simulink model "Appl_DrLearn_CtrlModel"  (R2018b)
settings: configuration reference "CodeConfig_10_ms" (kept outside this file)
undefined symbols (not defined in the file): CAL_LearnAllTimeMax_150s, CAL_LearnSingleTimeMax_60s, D_FirstMove, D_FourthlyMove, D_Invalid, D_SecondMove, D_ThirdlyMove, enDrAdjustEnable, FALSE, TRUE
libraries: DareLib x43, simulink x2
(part 2 of 2)

== stateflow chart Appl_DrLearn_CtrlModel/LogicCtrl/LocalAdjustCtrl/LearnReqDeal/Learn ==
  state [Hight,H_Move,Length,L_Move,Back,B_Move,Front,F_Move] = MotorLearnOrderPrm(VehicleTypePrm) [function] [commented out]
  state SetDescLearnStsForDebug(Sts) [function] [commented out]
  state SetDescLearnSts(Sts) [function]
  note: /*Hight,H_Move,Length,L_Move,Back,B_Move,Front,F_Move = MotorLearnOrderPrm(MtrCtrl_VehiclePrm);*/
  state Init
    en:
    SetDescLearnSts(FALSE);
    HeightLearnSW = enNULL;
    LengthLearnSW = enNULL;
    BackLearnSW = enNULL;
    FrontLearnSW = enNULL;;
    LearnResult = 0;
    MotorMtrCtrl_LearnSts = 0;
    Hight =D_FirstMove;
    H_Move =  enDOWN_BACK;
    Length =  D_SecondMove;
    L_Move = enUP_FORWARD;
    Back =  D_ThirdlyMove;
    B_Move = enUP_FORWARD;
    Front = D_FourthlyMove;
    F_Move = enUP_FORWARD;
  state LearnReady
    en:
    SetDescLearnSts(FALSE);
    HeightLearnSW = enNULL;
    LengthLearnSW = enNULL;
    BackLearnSW = enNULL;
    FrontLearnSW = enNULL;;
    LearnResult = 0;
    MotorMtrCtrl_LearnSts = 0;
    (default) -> (junction 223)
    LearnReady -> (junction 223) [order 1]
    (junction 223) -> (junction 225) [order 1] : [MtrCtrl_AdjustEnable == EN_DrTwelveWayMotor]
    (junction 223) -> (junction 229) [order 2]
    (junction 225) -> (junction 227) : {Hight =D_FirstMove;
        | H_Move =  enDOWN_BACK;
        | Length =  D_SecondMove;
        | L_Move = enUP_FORWARD;
        | Back =  D_ThirdlyMove;
        | B_Move = enUP_FORWARD;
        | Front = D_FourthlyMove;
        | F_Move = enUP_FORWARD;}
    (junction 227) -> (junction 229)
    (junction 229) -> (junction 232)
    (junction 232) -> (junction 234) [order 1] : [MtrCtrl_AdjustEnable == EN_DrSixWayMotor]
    (junction 232) -> (junction 238) [order 2]
    (junction 234) -> (junction 236) : {Hight =D_FirstMove;
        | H_Move =  enDOWN_BACK;
        | Length =  D_SecondMove;
        | L_Move = enUP_FORWARD;
        | Back =  D_ThirdlyMove;
        | B_Move = enUP_FORWARD;
        | Front = D_Invalid ;
        | F_Move = en_NULL;}
    (junction 236) -> (junction 238)
    (junction 238) -> (junction 241)
  state LearnLogicalDeal
    state HeightLearn
      en:
      HeightLearnSW = H_Move;
      LengthLearnSW = enNULL;
      BackLearnSW = enNULL;
      FrontLearnSW = enNULL;
      du:
      LearnAllRunTime++;
      HeightLearnTimer ++;
    state Learning
      en:
      LearnAllRunTime = 0;
      MotorMtrCtrl_LearnSts += 1;
      HeightLearnSW = enNULL;
      LengthLearnSW = enNULL;
      BackLearnSW = enNULL;
      FrontLearnSW =  enNULL;
      /*根据之前配置的电机动作顺序
      （1 2 3 4）查找动作顺序**/
    state LengthLearn
      en:
      HeightLearnSW = enNULL;
      LengthLearnSW = L_Move;
      BackLearnSW = enNULL;
      FrontLearnSW = enNULL;
      du:
      LearnAllRunTime++;
      LengthLearnTimer++;
    state BackLearn
      en:
      HeightLearnSW = enNULL;
      LengthLearnSW = enNULL;
      BackLearnSW = B_Move;
      FrontLearnSW = enNULL;
      du:
      LearnAllRunTime++;
      BackLearnTimer++;
    state FrontLearn
      en:
      HeightLearnSW = enNULL;
      LengthLearnSW = enNULL;
      BackLearnSW = enNULL;
      FrontLearnSW = F_Move;
      du:
      LearnAllRunTime++;
      FrontLearnTimer++;
    HeightLearn -> Learning : /*学习成功后记录当前的学习结果*/
        | [TRUE == MtrCtrl_HeightLockFault]
        | /LearnResult += MotorMtrCtrl_LearnSts ;
    Learning -> HeightLearn [order 1] : /*根据配置的设定顺序执行*/
        | [MotorMtrCtrl_LearnSts == Hight]
    LengthLearn -> Learning : [TRUE == MtrCtrl_LengthLockFault]
        | /LearnResult += MotorMtrCtrl_LearnSts;
    Learning -> LengthLearn [order 2] : [MotorMtrCtrl_LearnSts == Length]
    BackLearn -> Learning : [TRUE == MtrCtrl_BackLockFault]
        | /LearnResult += MotorMtrCtrl_LearnSts ;
    Learning -> BackLearn [order 4] : [MotorMtrCtrl_LearnSts == Back]
    FrontLearn -> Learning : [TRUE == MtrCtrl_FrontLockFault]
        | /LearnResult += MotorMtrCtrl_LearnSts ;
    Learning -> FrontLearn [order 3] : [MotorMtrCtrl_LearnSts == Front]
  (default) -> Init
  LearnReady -> Learning [order 2] : /*诊断请求自动学习*/
      | [hasChangedTo(MtrCtrl_DiagnoseLearnIn,TRUE)]
      | {LearnAllRunTime = 0;
      | HeightLearnTimer = 0;
      | LengthLearnTimer = 0;
      | BackLearnTimer = 0;
      | FrontLearnTimer = 0;
      | MtrCtrl_LearnSts = enLearnning;
      | LearnExitCause  = enInvalid;}
  Init -> LearnReady : /* 满足学习条件*/
      | [TRUE == LearnCondition]
  Learning -> LearnReady [order 5] : /*4个方向均学习完成后开始复位*/
      | [LearnResult == (Hight+Length+Back+Front)]
      | {MtrCtrl_LearnSts = enLearnAllSuccess;}
  LearnLogicalDeal -> LearnReady [order 2] : /*诊断退出*/
      | [hasChangedTo(MtrCtrl_DiagnoseLearnIn,FALSE )]
      | /LearnExitCause = enDescStop;
      | MtrCtrl_LearnSts = enLearnSts.enNULL;
  LearnLogicalDeal -> LearnReady [commented out] : /*学习时间超时*/
      | [LearnAllRunTime >CAL_LearnAllTimeMax_150s]
      | /LearnExitCause = enLearnOverTime;
  LearnLogicalDeal -> LearnReady [order 3] : /*高度电机运行超时*/
      | [HeightLearnTimer > CAL_LearnSingleTimeMax_60s]
      | /LearnExitCause = enMotorRunOverTime_H;
      | MtrCtrl_LearnSts = enLearnSts.enNULL;
  LearnReady -> Init [order 1] : /*学习条件不满足*/
      | [FALSE == LearnCondition]
      | /LearnExitCause  = LearnConditionExitCause;
  LearnLogicalDeal -> LearnReady [order 5] : /*纵向电机运行超时*/
      | [LengthLearnTimer > CAL_LearnSingleTimeMax_60s]
      | /LearnExitCause = enMotorRunOverTime_L;
      | MtrCtrl_LearnSts = enLearnSts.enNULL;
  LearnLogicalDeal -> LearnReady [order 6] : /*靠背电机运行超时*/
      | [BackLearnTimer > CAL_LearnSingleTimeMax_60s]
      | /LearnExitCause = enMotorRunOverTime_B;
      | MtrCtrl_LearnSts = enLearnSts.enNULL;
  LearnLogicalDeal -> LearnReady [order 7] : /*腿托电机运行超时*/
      | [FrontLearnTimer > CAL_LearnSingleTimeMax_60s]
      | /LearnExitCause = enMotorRunOverTime_F;
      | MtrCtrl_LearnSts = enLearnSts.enNULL;
  LearnLogicalDeal -> LearnReady [order 1] : [hasChanged(MtrCtrl_AdjustEnable)]
      | /LearnExitCause = enCfgW_ADJUST;
      | MtrCtrl_LearnSts = enLearnSts.enNULL;
  LearnLogicalDeal -> Init [order 4] : /*学习条件不满足*/
      | [FALSE == LearnCondition]
      | /LearnExitCause  = LearnConditionExitCause;
      | MtrCtrl_LearnSts = enLearnSts.enNULL;
  data: Hight function_output double size=1; H_Move function_output double size=1; Length function_output double size=1; L_Move function_output double size=1; Back function_output double size=1; B_Move function_output double size=1; Front function_output double size=1; F_Move function_output double size=1; VehicleTypePrm function_input double size=1; Sts function_input double size=1; Sts function_input; LearnConditionExitCause input; LearnCondition input; MtrCtrl_HeightLockFault input; MtrCtrl_LengthLockFault input; MtrCtrl_BackLockFault input; MtrCtrl_FrontLockFault input; MtrCtrl_DiagnoseLearnIn input; MtrCtrl_VehiclePrm input; HeightRunOverTimeFlag input; BackRunOverTimeFlag input; LengthRunOverTimeFlag input; FrontRunOverTimeFlag input; HeightLearnSW output Enum: enSWMoveCmd; LengthLearnSW output Enum: enSWMoveCmd; BackLearnSW output Enum: enSWMoveCmd; FrontLearnSW output Enum: enSWMoveCmd; Hight local uint8; Length local uint8; Back local uint8; H_Move local Enum: enSWMoveCmd; L_Move local double; B_Move local Enum: enSWMoveCmd; F_Move local Enum: enSWMoveCmd; TRUE parameter; FALSE parameter; LearnResult local uint8; MotorMtrCtrl_LearnSts local uint8; Front local uint8; MtrCtrl_LearnSts output Enum: enLearnSts; LearnExitCause output Enum: enLearnExitCause; MtrCtr_InCurrLearnSts input; CAL_LearnAllTimeMax_150s parameter; LearnAllRunTime local uint16; D_FirstMove parameter; D_Invalid parameter; D_SecondMove parameter; D_ThirdlyMove parameter; HeightLearnTimer local double; LengthLearnTimer local double; BackLearnTimer local double; FrontLearnTimer local double; CAL_LearnSingleTimeMax_60s parameter; D_FourthlyMove parameter; MtrCtrl_AdjustEnable input

== stateflow chart Appl_DrLearn_CtrlModel/LogicCtrl/LocalAdjustCtrl/LearnReqDeal/Learn/MotorLearnOrderPrm/Chart ==
  note: 车型：C62X、C52X…
      | 	0：P20车型
      | 	1：BM400车型
  (default) -> (junction 1)
  (junction 1) -> (junction 3) : [ /*1 == VehicleTypePrm*/]
  (junction 1) -> (junction 7) [commented out] : {Hight =D_FirstMove;
      | H_Move =  enDOWN_BACK;
      | Length = D_SecondMove;
      | L_Move = enUP_FORWARD;
      | Back =  D_ThirdlyMove;
      | B_Move = enDOWN_BACK;
      | Front = D_FourthlyMove;
      | F_Move = enUP_FORWARD;}
  (junction 3) -> (junction 5) : {Hight =D_Invalid;
      | H_Move =  en_NULL;
      | Length =  D_SecondMove;
      | L_Move = enUP_FORWARD;
      | Back =  D_FirstMove;
      | B_Move = enUP_FORWARD;
      | Front = D_ThirdlyMove;
      | F_Move = enUP_FORWARD;}
  (junction 5) -> (junction 7)
  (junction 7) -> (junction 10)
  data: VehicleTypePrm input; Hight output double; H_Move output Enum: enSWMoveCmd; Length output double; L_Move output Enum: enSWMoveCmd; Back output double; B_Move output Enum: enSWMoveCmd; Front output double; F_Move output Enum: enSWMoveCmd; D_FirstMove parameter; D_FourthlyMove parameter; D_Invalid parameter; D_ThirdlyMove parameter; D_SecondMove parameter
